simulink model "TPEtape1simulink"  (R2025b)
settings: Solver=VariableStepAuto  StartTime=0.0  StopTime=2000  RelTol=1e-3
values from neighbouring files (symbols this model uses):
  K1 = 0.02    [Partie1TPauto.m]    (also in Partie2TPauto.m; Partie3TPauto.m)
  K2 = 5 * 10^(-3)    (= 0.005)    [Partie1TPauto.m]    (also in Partie2TPauto.m; Partie3TPauto.m)
  tau1 = 2000    [Partie1TPauto.m]    (also in Partie2TPauto.m; Partie3TPauto.m)
  tau2 = 2    [Partie1TPauto.m]    (also in Partie2TPauto.m)
settings Model: Creator=dayan  LastModifiedBy=dayan

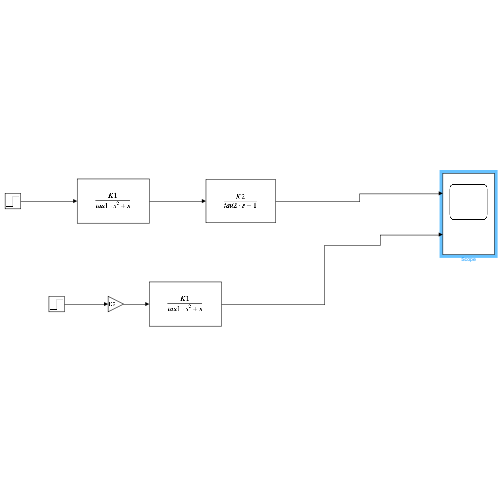
[thumbnail: Simulink's stored preview of the top-level diagram]
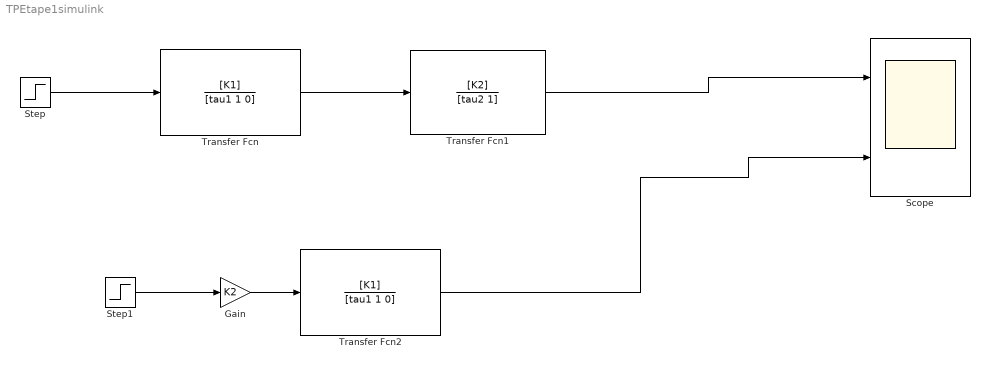
== system TPEtape1simulink ==
  Gain : Gain  Gain=K2
  Scope : Scope  NumInputPorts=2
      settings: Title=coucou petasse  ActiveDisplayYMinimum=-0.00918908567211559  ActiveDisplayYMaximum=0.082701771049040335  YLabel=Amplitude
  Step : Step  SampleTime=0
  Step1 : Step  SampleTime=0
  Transfer Fcn : TransferFcn  Numerator=[K1]  Denominator=[tau1 1 0]
  Transfer Fcn1 : TransferFcn  Numerator=[K2]  Denominator=[tau2 1]
  Transfer Fcn2 : TransferFcn  Numerator=[K1]  Denominator=[tau1 1 0]
  wires:
  Step/1 -> Transfer Fcn/1
  Transfer Fcn/1 -> Transfer Fcn1/1
  Transfer Fcn1/1 -> Scope/1
  Step1/1 -> Gain/1
  Gain/1 -> Transfer Fcn2/1
  Transfer Fcn2/1 -> Scope/2
